simulink model "LGR"  (R2024a)
settings: Solver=VariableStepAuto  StartTime=0.0  StopTime=25  RelTol=1e-3
model workspace (MAT data in the model file):
  g = 9.81
  l = 3.7
values from neighbouring files (symbols this model uses):
  A = [0 1 0; 0 0 1; 0 -g/l 0]    [LGRgains.m]
  B = [0 0 1]'    [LGRgains.m]
  C = [g/l 0 0]    [LGRgains.m]
  K_i = K_q(end)    [LGRgains.m]
  K_x = K_q(1:(end-1))    [LGRgains.m]
  L = place(A', C', ePoles)'    [LGRgains.m]
settings Model: Creator=Riley  LastModifiedBy=Riley

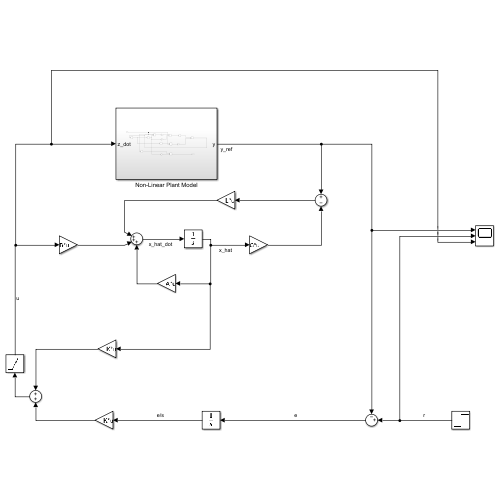
[thumbnail: Simulink's stored preview of the top-level diagram]
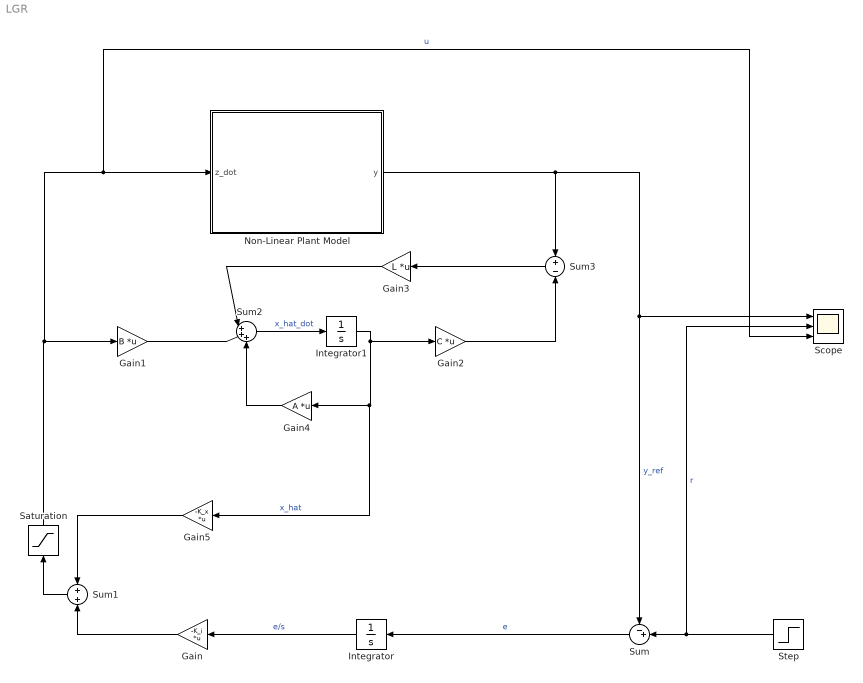
== system LGR ==
  Gain : Gain  Gain=-K_i  Multiplication=Matrix(K*u)
  Gain1 : Gain  Gain=B  Multiplication=Matrix(K*u)
  Gain2 : Gain  Gain=C  Multiplication=Matrix(K*u)
  Gain3 : Gain  Gain=L  Multiplication=Matrix(K*u)
  Gain4 : Gain  Gain=A  Multiplication=Matrix(K*u)
  Gain5 : Gain  Gain=-K_x  Multiplication=Matrix(K*u)
  Integrator : Integrator
  Integrator1 : Integrator
  Non-Linear Plant Model : Subsystem
  Saturation : Saturate  UpperLimit=1  LowerLimit=-1
  Scope : Scope  NumInputPorts=3
  Step : Step  Time=0  SampleTime=0
  Sum : Sum  Inputs=-+|
  Sum1 : Sum  Inputs=+|+
  Sum2 : Sum  Inputs=|+++
  Sum3 : Sum  Inputs=+|-
  wires:
  Step/1 -> Scope/2, Sum/2  "r"
  Non-Linear Plant Model/1(y) -> Sum3/1, Sum/1, Scope/1  "y_ref"
  Sum/1 -> Integrator/1  "e"
  Integrator/1 -> Gain/1  "e/s"
  Gain/1 -> Sum1/2
  Sum1/1 -> Saturation/1
  Gain1/1 -> Sum2/2
  Sum2/1 -> Integrator1/1  "x_hat_dot"
  Integrator1/1 -> Gain5/1, Gain4/1, Gain2/1  "x_hat"
  Gain2/1 -> Sum3/2
  Sum3/1 -> Gain3/1
  Gain3/1 -> Sum2/1
  Gain4/1 -> Sum2/3
  Gain5/1 -> Sum1/1
  Saturation/1 -> Gain1/1, Scope/3, Non-Linear Plant Model/1(z_dot)  "u"

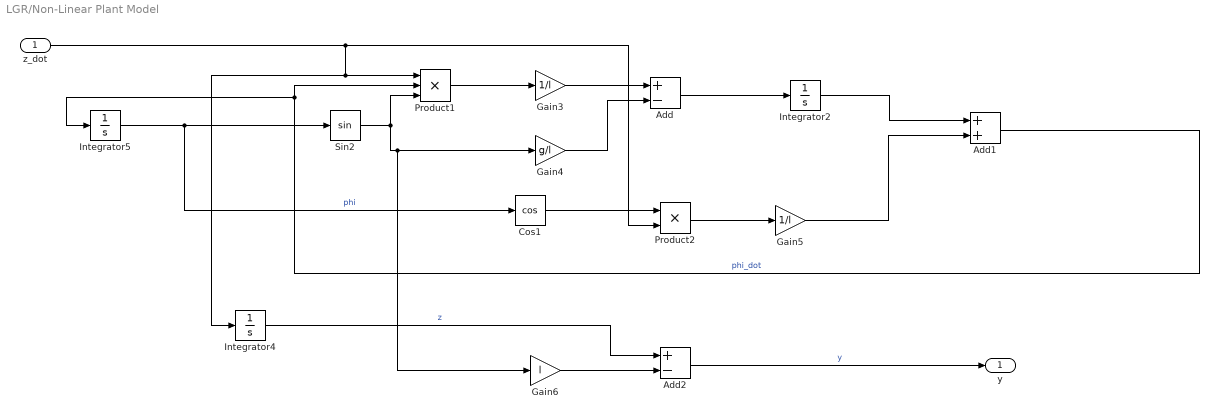
== system LGR/Non-Linear Plant Model ==
  z_dot : Inport
  Add : Sum  Inputs=+-
  Add1 : Sum
  Add2 : Sum  Inputs=+-
  Cos1 : Trigonometry  Operator=cos
  Gain3 : Gain  Gain=1/l
  Gain4 : Gain  Gain=g/l
  Gain5 : Gain  Gain=1/l
  Gain6 : Gain  Gain=l
  Integrator2 : Integrator
  Integrator4 : Integrator
  Integrator5 : Integrator
  Product1 : Product  Inputs=3
  Product2 : Product
  Sin2 : Trigonometry
  y : Outport
  wires:
  z_dot/1 -> Integrator4/1, Product1/1, Product2/2
  Sin2/1 -> Gain4/1, Gain6/1, Product1/3
  Product1/1 -> Gain3/1
  Add1/1 -> Product1/2, Integrator5/1  "phi_dot"
  Gain3/1 -> Add/1
  Integrator5/1 -> Cos1/1, Sin2/1  "phi"
  Integrator2/1 -> Add1/1
  Add/1 -> Integrator2/1
  Cos1/1 -> Product2/1
  Product2/1 -> Gain5/1
  Gain4/1 -> Add/2
  Gain5/1 -> Add1/2
  Gain6/1 -> Add2/2
  Integrator4/1 -> Add2/1  "z"
  Add2/1 -> y/1  "y"
